simulink model "local_noise"  (R2023a)
settings: Solver=VariableStepAuto  StartTime=0.0  StopTime=10  RelTol=1e-3
values from neighbouring files (symbols this model uses):
  A0 = Ai-Bi*K0    [Project_globale.m]    (also in Project_locale.m)
  Ad = [0 0 0 0 0 0 ... (first row only)    [Project_globale.m]    (also in Project_locale.m)
  Ai = A0    [Project_globale.m]    (also in Project_locale.m)
  Bi = [ 0 ; -9.9453]    [Project_globale.m]    (also in Project_locale.m)
  c = 10/2*min(real(lambda_g))    [Project_globale.m]    (also in Project_locale.m)
  Ci = [708.27 0]    [Project_globale.m]    (also in Project_locale.m)
  D0 = 0    [Project_globale.m]    (also in Project_locale.m)
  Di = zeros(1,2)    [Project_globale.m]    (also in Project_locale.m)
  F1 = place(Ai',-c*Ci',[-1 -2])'    [Project_locale.m]
  G = diag([1 0 0 0 0 0])    [Project_globale.m]    (also in Project_locale.m)
  K = R^-1*Bi'*P    [Project_globale.m]    (also in Project_locale.m)
  x0 = [3,1]    [Project_globale.m]    (also in Project_locale.m)
settings Model: Creator=Giulia  LastModifiedBy=Giulia

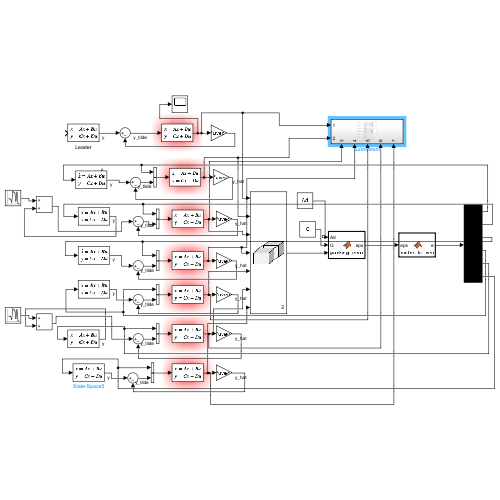
[thumbnail: Simulink's stored preview of the top-level diagram]
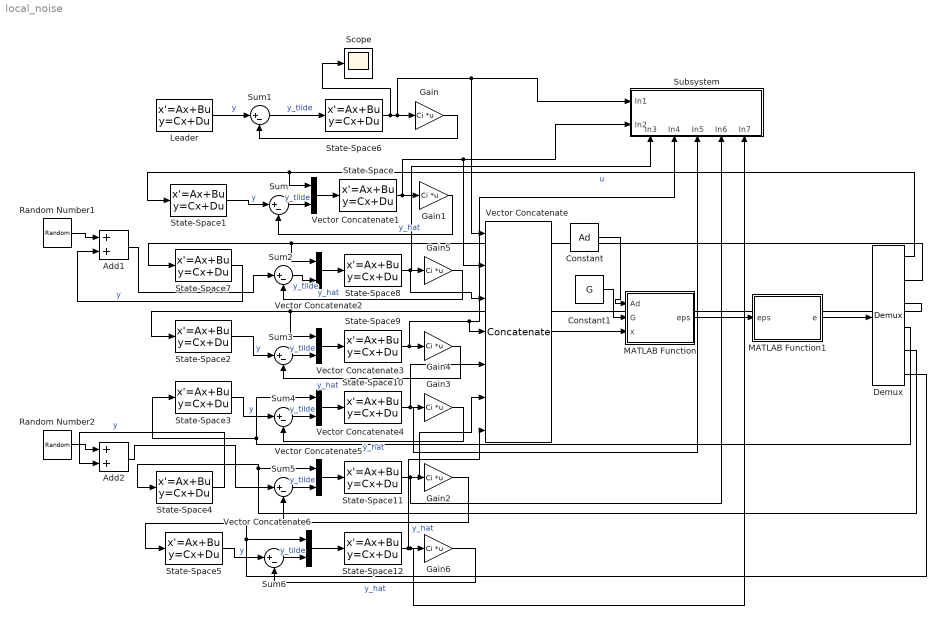
== system local_noise ==
  Add1 : Sum
  Add2 : Sum
  Constant : Constant  Value=Ad
  Constant1 : Constant  Value=G
  Demux : Demux  Outputs=size(Ad,1)
  Gain{,1..6} (7 alike) : Gain  Gain=Ci  Multiplication=Matrix(K*u) (u vector)
  Leader : StateSpace  A=A0  B=Bi  C=Ci  D=D0  InitialCondition=x0
  MATLAB Function : MATLAB Function  TreatAsAtomicUnit=on
  MATLAB Function1 : MATLAB Function  TreatAsAtomicUnit=on
  Random Number1 : RandomNumber  Variance=10000  SampleTime=0.1
  Random Number2 : RandomNumber  Variance=10000  SampleTime=0.1
  Scope : Scope
  State-Space{,8..12} (6 alike) : StateSpace  A=Ai  B=[c*Bi*K, -c*F1]  C=eye(2)  D=zeros(2,3)  InitialCondition=x0
  State-Space1 : StateSpace  A=Ai  B=c*Bi*K  C=Ci  D=Di  InitialCondition=x0  ParameterTunability=Optimized
  State-Space{2..5,7} (5 alike) : StateSpace  A=Ai  B=c*Bi*K  C=Ci  D=Di  InitialCondition=x0
  State-Space6 : StateSpace  A=Ai  B=-c*F1  C=eye(2)  D=zeros(2,1)  InitialCondition=x0
  Subsystem : Subsystem
      settings: PortSchema="{\"entries\":[{\"content\":{\"sides\":[{\"content\":{\"connectorIds\":[\"In1\",\"In2\"]},\"type\":\"ConnectorPlacement.EquallySpacedRectSide\",\"uuid\":\"e5690f60-dfa3-4d24-845c-eb19d446c7ee\"},{\"content\":{\"side\":\"RIGHT\"},\"type\":\"ConnectorPlacement.EquallySpacedRectSide\",\"uuid\":\"a41d9e4a-267d-44ba-a380-b8d8ea4e3cb9\"},{\"content\":{\"side\":\"TOP\"},\"type\":\"ConnectorPlacement.EquallySpacedRectSide\",\"uuid\":\"990e4c72-4654-4e9a-98e4-634db6676fa3\"},{\"content\":{\"connectorIds\":[\"In3\",\"In4\",\"In5\",\"In6\",\"In7\"],\"side\":\"BOTTOM\"},\"type\":\"ConnectorPlacement.EquallySpacedRectSide\",\"uuid\":\"e75a7693-b495-4998-ab10-28f33e3d4652\"}]},\"type\":\"ConnectorPlacement.EquallySpacedConnector\",\"uuid\":\"cc17a25f-dba8-4ee4-98f7-88763bf16359\"}],\"packageUris\":[\"http://schema.mathworks.com/mf0/Connector/R2020b\"],\"version\":\"1.0\"}"
  Sum{,1..6} (7 alike) : Sum  Inputs=|+-
  Vector Concatenate : Concatenate  NumInputs=7  Mode=Multidimensional array  ConcatenateDimension=2
  Vector Concatenate{1..6} (6 alike) : Concatenate
  wires:
  Gain2/1 -> Sum5/2  "y_hat"
  Demux/4 -> State-Space3/1, Vector Concatenate4/1
  Gain6/1 -> Sum6/2  "y_hat"
  Gain1/1 -> Sum/2  "y_hat"
  Demux/6 -> State-Space5/1, Vector Concatenate6/1
  State-Space12/1 -> Subsystem/7(In7), Gain6/1, Vector Concatenate/7
  Gain/1 -> Sum1/2
  Sum4/1 -> Vector Concatenate4/2  "y_tilde"
  State-Space10/1 -> Vector Concatenate/5, Subsystem/5(In5), Gain3/1
  Sum/1 -> Vector Concatenate1/2  "y_tilde"
  Demux/2 -> State-Space7/1, Vector Concatenate2/1
  State-Space11/1 -> Subsystem/6(In6), Vector Concatenate/6, Gain2/1
  Gain4/1 -> Sum3/2  "y_hat"
  Gain5/1 -> Sum2/2  "y_hat"
  Vector Concatenate5/1 -> State-Space11/1
  Vector Concatenate/1 -> MATLAB Function/3(x)
  State-Space6/1 -> Scope/1, Gain/1, Subsystem/1(In1), Vector Concatenate/1
  Vector Concatenate4/1 -> State-Space10/1
  MATLAB Function1/1(e) -> Demux/1
  Gain3/1 -> Sum4/2  "y_hat"
  Demux/3 -> Vector Concatenate3/1, State-Space2/1
  State-Space8/1 -> Vector Concatenate/3, Subsystem/3(In3), Gain5/1
  Sum5/1 -> Vector Concatenate5/2  "y_tilde"
  Sum2/1 -> Vector Concatenate2/2  "y_tilde"
  Sum6/1 -> Vector Concatenate6/2  "y_tilde"
  Constant1/1 -> MATLAB Function/2(G)
  Vector Concatenate1/1 -> State-Space/1
  Vector Concatenate2/1 -> State-Space8/1
  Demux/5 -> Vector Concatenate5/1, State-Space4/1
  MATLAB Function/1(eps) -> MATLAB Function1/1(eps)
  Constant/1 -> MATLAB Function/1(Ad)
  Sum3/1 -> Vector Concatenate3/2  "y_tilde"
  State-Space9/1 -> Vector Concatenate/4, Subsystem/4(In4), Gain4/1
  Vector Concatenate3/1 -> State-Space9/1
  Vector Concatenate6/1 -> State-Space12/1
  Demux/1 -> Vector Concatenate1/1, State-Space1/1  "u"
  State-Space/1 -> Subsystem/2(In2), Vector Concatenate/2, Gain1/1
  Sum1/1 -> State-Space6/1  "y_tilde"
  State-Space1/1 -> Sum/1  "y"
  State-Space2/1 -> Sum3/1  "y"
  State-Space3/1 -> Sum4/1  "y"
  Add1/1 -> Sum2/1
  State-Space7/1 -> Add1/2  "y"
  Random Number1/1 -> Add1/1
  Leader/1 -> Sum1/1  "y"
  State-Space5/1 -> Sum6/1  "y"
  Random Number2/1 -> Add2/1
  Add2/1 -> Sum5/1
  State-Space4/1 -> Add2/2  "y"

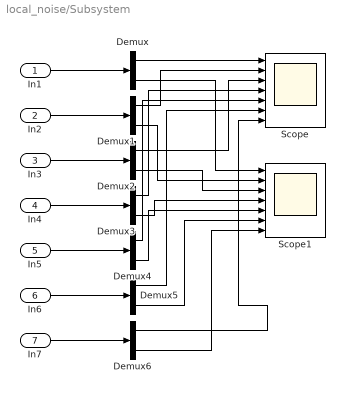
== system local_noise/Subsystem ==
  In1 : Inport
  In2 : Inport  Port=2
  In3 : Inport  Port=3
  In4 : Inport  Port=4
  In5 : Inport  Port=5
  In6 : Inport  Port=6
  In7 : Inport  Port=7
  Demux{,1..6} (7 alike) : Demux  Outputs=2
  Scope : Scope  NumInputPorts=7
  Scope1 : Scope  NumInputPorts=7
  wires:
  In1/1 -> Demux/1
  In2/1 -> Demux1/1
  In3/1 -> Demux2/1
  In4/1 -> Demux3/1
  In5/1 -> Demux4/1
  In6/1 -> Demux5/1
  In7/1 -> Demux6/1
  Demux/1 -> Scope/1
  Demux1/1 -> Scope/2
  Demux2/1 -> Scope/3
  Demux3/1 -> Scope/4
  Demux4/1 -> Scope/5
  Demux5/1 -> Scope/6
  Demux6/1 -> Scope/7
  Demux/2 -> Scope1/1
  Demux1/2 -> Scope1/2
  Demux2/2 -> Scope1/3
  Demux3/2 -> Scope1/4
  Demux4/2 -> Scope1/5
  Demux5/2 -> Scope1/6
  Demux6/2 -> Scope1/7

== matlab function local_noise/MATLAB Function1 ==
  data: eps input; e output
function e = matrix_to_vec(eps)

e=zeros(size(eps,1)*size(eps,2),1);
for i=1:size(eps,2)
    for j=1:size(eps,1)
        e((i-1)*size(eps,1)+j)=eps(j,i);
    end
end

== matlab function local_noise/MATLAB Function ==
  data: Ad input; G input; eps output; x input
function eps = tracking_error(Ad, G, x)

eps=zeros(size(x,1),size(Ad,1));            %2 righe, 6 colonne
for i=1:size(Ad,1)
    sum=zeros(2,1);
    for j=1:size(Ad,1)
        sum=sum+Ad(i,j)*(x(:,1+j)-x(:,1+i));
    end
    sum=sum+G(i,i)*(x(:,1)-x(:,1+i));
    eps(:,i)=sum;
end
